simulink model "ExampleDemo3"  (Simulink 5.0)
settings: Solver=ode45  StartTime=0.0  StopTime=2.0  RelTol=1e-3
values from neighbouring files (symbols this model uses):
  den = [1]    [dab1.m]    (also in dab1o.m)
  dx = 0    [dab1.m]    (also in dab1o.m)
  num = [1]    [dab1.m]    (also in dab1o.m)
undefined symbols (not defined in the file or in its folder): get
libraries: simulink x1, dspsnks4 x1
settings Model: LastModifiedBy=Praveen

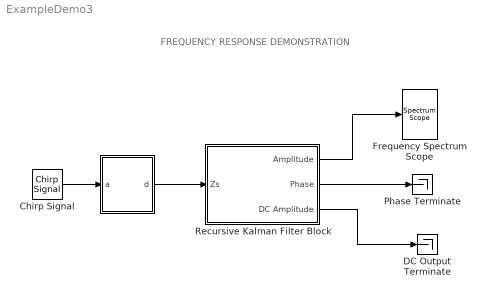
== system ExampleDemo3 ==
  note: FREQUENCY RESPONSE DEMONSTRATION
  "  " : Subsystem  mask(Data Adquisition Board){filter=on, approx=Butterworth, order=3, numerator=[], denominator=[], freq=180, resdis=on, vertres=8, xmax=100, winsize=1, G=1.0, fs=60*32}
      mask prompts: filter "Disable Analog Filter"; approx "Filter approximation"; numerator "Free expression filter: numerator(descending order of s)"; denominator "Free expression filter: denominator:"; freq "Cut-off frequency"; resdis "Disable Vertical Resolution"; vertres "Vertical Resolution: No. of bits"; xmax "Vertical Resolution: signal range"; winsize "Window size"; G "Gain"; fs "Sampling frequency"
      mask help: Takes the instantaneous value of the input signal and convert it to the data window of samples.
      mask init:
      | dab1
      mask Help: web(['file:///' which('dab.html')]);
      mask StyleString: checkbox,popup(Bessel|Tschebyscheff|Butterworth|free expression),popup(2|3|4),edit,edit,edit,checkbox,popup(8|12|16),edit,edit,edit,edit
      mask Display: disp('DAB')
  Chirp Signal : simulink/Sources/Chirp Signal  f1=0  T=3  f2=300  VectorParams1D=off
  DC Output Terminate : Terminator
  Frequency Spectrum Scope : dspsnks4/Spectrum Scope  ScopeProperties=off  Domain=Frequency  HorizSpan=1  UseBuffer=on  BufferSize=128  Overlap=64  inpFftLenInherit=on  FFTlength=128  numAvg=2  DisplayProperties=off  AxisGrid=on  Memory=on  FrameNumber=off  AxisLegend=off  AxisZoom=off  OpenScopeAtSimStart=on  OpenScopeImmediately=off  FigPos=get(0,'defaultfigureposition')  AxisProperties=on  XUnits=Hertz  XRange=[0...Fs/2]  InheritXIncr=on  XIncr=1.0  XLabel=Samples  YUnits=dB  YLabel=Magnitude, dB  LineProperties=off  LineStyles=-  LineMarkers=None  LineColors=[1 0 0]
      settings: YMin=-40  YMax=5
  Phase Terminate : Terminator
  Recursive Kalman Filter Block : Subsystem  mask(Kalman Block){f=60, Fs=32, X0=[0;0;0], C=[1 0 1], sigman=0.01, sigmav=0.005, M=[(0.24^2) 0 0;0 (0.24^2) 0;0 0 (0.24^2)], lambda=1000}
      mask prompts: f "Fundamental Frequency of Input Signal (f) in Hz"; Fs "Sampling Frequency (Fs) in samples per second"; X0 "Initial State (x0)"; C "Voltage-Phasor relation matrix (C)"; sigman "Measurement Noise Variance (Sigma n)"; sigmav "Process noise variance (Sigma v)"; M "Single step transition error covariance (M)"; lambda "Decaying DC Parameter (lambda)"
      mask help:
      | Measures the Phasor voltage values using the Kalman filter.
      | The input to the block is 'Zs(n)', the signal at time nT. 'f' is the fundamental frequency of the signal, and the harmonics are assumed to be integral multiple of this.
      | 'C' is the ralationship between voltage and phasor values. The default value is [1,0,1] assuming zero imaginary component and non-zero DC component.
      | Measurement noise variance 'sigman' models the noise during the voltage measurement.
      | Process variance 'sigmav' denotes the variation in the measurement of voltage values.
      | 'M' denotes the single step variation
      | Decaying DC component models the decreasing nature of the DC.
  wires:
  Chirp Signal/1 -> "  "/1(a)
  "  "/1(d) -> Recursive Kalman Filter Block/1(Zs)
  Recursive Kalman Filter Block/1(Amplitude) -> Frequency Spectrum Scope/1
  Recursive Kalman Filter Block/3(DC Amplitude) -> DC Output Terminate/1
  Recursive Kalman Filter Block/2(Phase) -> Phase Terminate/1

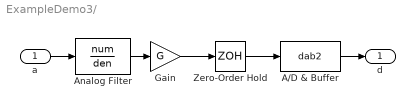
== system ExampleDemo3/   ==
  a : Inport
  A/D & Buffer : S-Function  FunctionName=dab2  Parameters=winsize,fs,dx,resdis
  Analog Filter : TransferFcn  Numerator=num  Denominator=den
  Gain : Gain  Gain=G  SaturateOnIntegerOverflow=on
  Zero-Order Hold : ZeroOrderHold  SampleTime=1/fs
  d : Outport  InitialOutput=[zeros(winsize,1)]
  wires:
  A/D & Buffer/1 -> d/1
  a/1 -> Analog Filter/1
  Zero-Order Hold/1 -> A/D & Buffer/1
  Gain/1 -> Zero-Order Hold/1
  Analog Filter/1 -> Gain/1

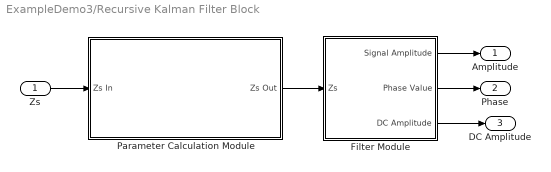
== system ExampleDemo3/Recursive Kalman Filter Block ==
  Zs : Inport
  Filter Module : Subsystem  Priority=2
  Parameter Calculation Module : Subsystem  Priority=1
      mask Display:
      | disp('PARAMETER MODULE');
      | port_label('input',1,'Zs in');
      | port_label('output',1,'Zs out');
  Amplitude : Outport
  Phase : Outport  Port=2
  DC Amplitude : Outport  Port=3
  wires:
  Zs/1 -> Parameter Calculation Module/1(Zs In)
  Parameter Calculation Module/1(Zs Out) -> Filter Module/1(Zs)
  Filter Module/1(Signal Amplitude) -> Amplitude/1
  Filter Module/3(DC Amplitude) -> DC Amplitude/1
  Filter Module/2(Phase Value) -> Phase/1

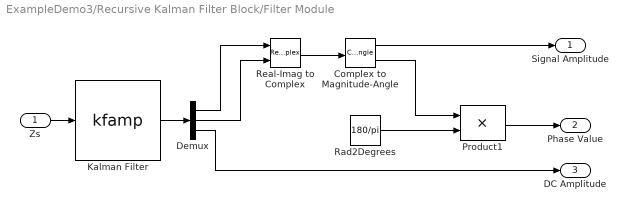
== system ExampleDemo3/Recursive Kalman Filter Block/Filter Module ==
  Zs : Inport
  Complex to Magnitude-Angle : ComplexToMagnitudeAngle
  Demux : Demux  Outputs=3
  Kalman Filter : S-Function  Priority=2  FunctionName=kfamp  Parameters=X0 C M
      mask Type: Kalman Filter Block
  Product1 : Product  ShowAdditionalParam=on  SaturateOnIntegerOverflow=on
  Rad2Degrees : Constant  Value=180/pi
  Real-Imag to Complex : RealImagToComplex
  Signal Amplitude : Outport
  Phase Value : Outport  Port=2
  DC Amplitude : Outport  Port=3
  wires:
  Zs/1 -> Kalman Filter/1
  Kalman Filter/1 -> Demux/1
  Demux/1 -> Real-Imag to Complex/1
  Demux/2 -> Real-Imag to Complex/2
  Demux/3 -> DC Amplitude/1
  Product1/1 -> Phase Value/1
  Real-Imag to Complex/1 -> Complex to Magnitude-Angle/1
  Complex to Magnitude-Angle/1 -> Signal Amplitude/1
  Rad2Degrees/1 -> Product1/2
  Complex to Magnitude-Angle/2 -> Product1/1

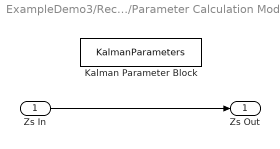
== system ExampleDemo3/Recursive Kalman Filter Block/Parameter Calculation Module ==
  Zs In : Inport
  Kalman Parameter Block : S-Function  Priority=1  FunctionName=KalmanParameters  Parameters=Fs f sigman sigmav M lambda
  Zs Out : Outport
  wires:
  Zs In/1 -> Zs Out/1
